simulink model "model_schuettgut"  (R2020a)
settings: Solver=VariableStepAuto  StartTime=0.0  StopTime=600  MaxStep=1e-2  MinStep=1e-5  RelTol=1e-2
libraries: simulink x8, library_schuettgut x5
settings Model: Creator=Jonathan  LastModifiedBy=Jonathan
settings DataIOCC: SaveState=on

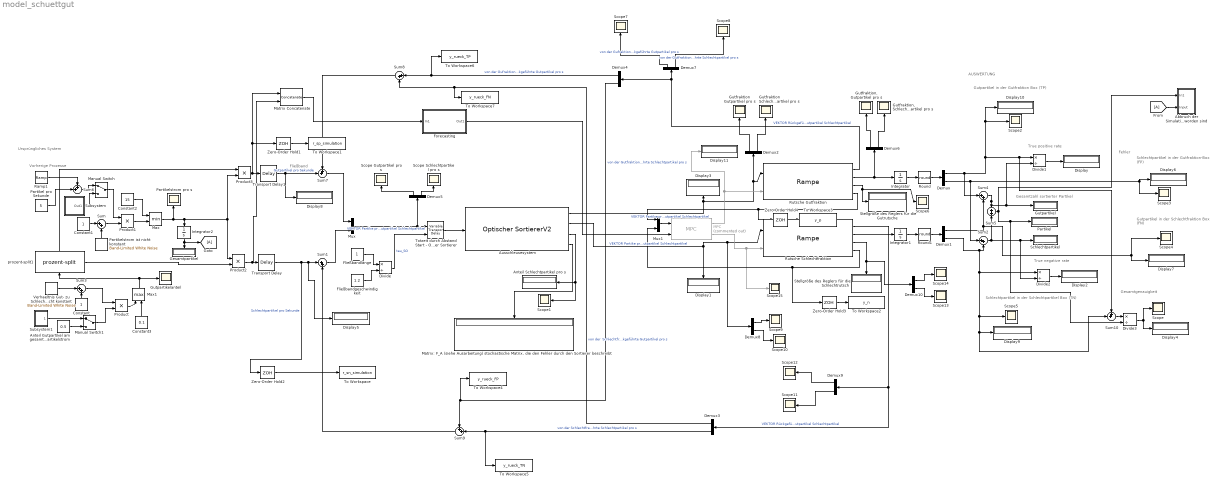
== system model_schuettgut ==
  note: Fließband
  note: Vorherige Prozesse
  note: Gesamtgenauigkeit
  note: True negative rate
  note: Gutpartikel in der
      | Schlechtfraktion Box (FN)
  note: Schlechtpartikel in der
      | Gutfraktion-Box (FP)
  note: Schlechtpartikel in der
      | Schlechtpartikel Box (TN)
  note: AUSWERTUNG
  note: True positive rate
  note: Gesamtzahl sortierter Partikel
  note: Gutpartikel in der
      | Gutfraktion Box (TP)
  note: Fehler
  note: Ursprüngliches System
  Abbruch der Simulation sobald alle Partikel sortiert worden sind : Subsystem
  Anteil Gutpartikel am gesamten Partikelstrom : Constant  Value=0.5
  Anteil Schlechtpartikel pro s : Display
  Ausschleusesystem : library_schuettgut/Optischer SortiererV2  alpha=0.04  beta=0.05
  Constant : Constant
  Constant1 : Constant
  Constant2 : Constant  Value=15
  Constant3 : Constant  Value=0.1
  Demux{,1..10} (11 alike) : Demux  Outputs=2
  Display{,1..11} (12 alike) : Display
  Divide{,1..3} (4 alike) : Product  Inputs=*/
  Fließbandgeschwindigkeit : Constant  Value=1.2
  Fließbandlänge : Constant
  Forecasting : Subsystem
  Gesamtpartikel : Display
  Gutfraktion Gutpartikel pro s : Scope
  Gutfraktion Schlechtpartikel pro s : Scope
  "Gutfraktion, Gutpartikel pro s" : Scope
  "Gutfraktion, Schlechtpartikel pro s" : Scope
  Gutpartikel : Display
  Gutpartikelanteil : Scope
  Integrator : Integrator
  Integrator1 : Integrator
  Integrator2 : Integrator
  MPC : library_schuettgut/MPC  Commented=on  SystemSampleTime=-1  Latency=0  AutoFrameSizeCalculation=off
      link override Constant: Value=12
      link override Constant2: Value=1
      link override Constant3: Value=4
      link override Constant4: Value=20
      link override Constant5: Value=8
      link override Constant6: Value=zeros(4,12)
  Manual Switch : ManualSwitch
  Manual Switch1 : ManualSwitch
  Matrix Concatenate : Concatenate  Mode=Multidimensional array  ConcatenateDimension=2
  "Matrix: F_A (siehe Ausarbeitung) stochastische Matrix, die den Fehler durch den Sortierer beschreibt" : Display
  Max : MinMax  Inputs=2
  Max1 : MinMax  Function=max  Inputs=2
  Mux : Mux  Inputs=2
  Mux1 : Mux  Inputs=2
  Partikel : Display
  Partikel pro Sekunde : Constant  Value=5
  Partikelstrom ist nicht konstant : simulink/Sources/Band-Limited White Noise  Cov=[0.00001]  Ts=0.1  seed=[23341]
  Partikelstrom pro s : Scope
  Product{,1..3} (4 alike) : Product
  Ramp1 : simulink/Sources/Ramp  slope=0.01  start=200  InitialOutput=0
  Round : Rounding  Operator=round
  Round1 : Rounding  Operator=round
  Rutsche Gutfraktion : library_schuettgut/Rampe  Tag=Rampe  OK=2  errorP=0  errorN=0  KV=0.2  V=1  TrueorFalse=0  delay=0.2  gain=8.6  KP=0  KN=0
  Rutsche Schlechtfraktion : library_schuettgut/Rampe  Tag=Rampe  OK=2  errorP=0  errorN=0  KV=0.2  V=1  TrueorFalse=1  delay=0.2  gain=0  KP=0  KN=0
  Schlechtpartikel : Display
  Scope{,1..15} (16 alike) : Scope
  Scope Gutpartikel pro s : Scope
  Scope Schlechtpartikel pro s : Scope
  Stellgröße des Reglers für die Gutrutsche : Display
  Stellgröße des Reglers für die Schlechtrutsch : Display
  Subsystem : Subsystem
  Subsystem1 : Subsystem
  Sum{,1..4,8} (6 alike) : Sum  Inputs=|++
  Sum{6..7,9..10} (4 alike) : Sum  Inputs=++|
  Sum5 : Sum  Inputs=+|+
  To Workspace : ToWorkspace  VariableName=r_sn_simulation  SaveFormat=Timeseries  SampleTime=-1
  To Workspace1 : ToWorkspace  VariableName=r_sp_simulation  SaveFormat=Timeseries  SampleTime=-1
  To Workspace2 : ToWorkspace  VariableName=y_n  SaveFormat=Timeseries  SampleTime=-1
  To Workspace3 : ToWorkspace  VariableName=y_p  SaveFormat=Timeseries  SampleTime=-1
  To Workspace4 : ToWorkspace  VariableName=y_rueck_FP  SaveFormat=Timeseries  SampleTime=0.1
  To Workspace5 : ToWorkspace  VariableName=y_rueck_TN  SaveFormat=Timeseries  SampleTime=0.1
  To Workspace6 : ToWorkspace  VariableName=y_rueck_TP  SaveFormat=Timeseries  SampleTime=0.1
  To Workspace7 : ToWorkspace  VariableName=y_rueck_FN  SaveFormat=Timeseries  SampleTime=0.1
  Totzeit durch Abstand Start - Optischer Sortierer : VariableTransportDelay  VariableDelayType=Variable transport delay  MaximumDelay=10  MaximumPoints=30000
  Transport Delay : TransportDelay  DelayTime=160  BufferSize=4096
  Transport Delay1 : TransportDelay  DelayTime=160  BufferSize=2048
  Verhaeltnis Gut- zu Schlechtpartikel ist nicht konstant : simulink/Sources/Band-Limited White Noise  Cov=[0.00001]  Ts=0.1  seed=[13341]
  Zero-Order Hold{1..4} (4 alike) : ZeroOrderHold  SampleTime=0.1
  prozent-split1 : library_schuettgut/prozent-split  SystemSampleTime=-1  Latency=0  AutoFrameSizeCalculation=off
      settings: PortSchema="{\"entries\":[{\"content\":{\"sides\":[{\"content\":{\"connectorIds\":[\"In1\"]},\"type\":\"ConnectorPlacement.EquallySpacedRectSide\",\"uuid\":\"ab8511c8-9f1d-48ad-bf24-85fd477f0bdd\"},{\"content\":{\"connectorIds\":[\"Out1\"],\"side\":\"RIGHT\"},\"type\":\"ConnectorPlacement.EquallySpacedRectSide\",\"uuid\":\"9ac1a19a-8176-444e-9f4d-7beffa0184e3\"},{\"content\":{\"connectorIds\":[\"Out2\"],\"side\":\"TOP\"},\"type\":\"ConnectorPlacement.EquallySpacedRectSide\",\"uuid\":\"376c2400-f821-4649-ab16-706a2da6117b\"}]},\"type\":\"ConnectorPlacement.EquallySpacedConnector\",\"uuid\":\"f6e72b2d-0467-4732-a018-d51f3a5db703\"}],\"packageUris\":[\"http://schema.mathworks.com/mf0/Connector/19700101\"],\"version\":\"1.0\"}"
  wires:
  Anteil Gutpartikel am gesamten Partikelstrom/1 -> Manual Switch1/2
  Max/1 -> Partikelstrom pro s/1, Integrator2/1, Product2/1, Product3/2
  Transport Delay1/1 -> Display8/1, Sum7/2  "Gutpartikel pro Sekunde"
  Totzeit durch Abstand Start - Optischer Sortierer/1 -> Ausschleusesystem/1
  Rutsche Gutfraktion/1 -> Demux4/1, Demux7/1  "VEKTOR Rückgeführte Partikel Gutfraktion pro s Gutpartikel Schlechtpartikel"
  Mux/1 -> Totzeit durch Abstand Start - Optischer Sortierer/1, Demux5/1  "VEKTOR Partike pro s: Gutpartikel Schlechtpartikel"
  Demux4/1 -> To Workspace6/1, Sum8/1  "von der Gufraktion zurückgeführte Gutpartikel pro s"
  Sum8/1 -> Sum7/1
  Sum9/1 -> Sum1/2
  Rutsche Gutfraktion/2 -> Demux6/1, Integrator/1
  Ausschleusesystem/1 -> Demux2/1, Rutsche Gutfraktion/1, Display3/1  "VEKTOR Partike pro s in der Gutfraktion: Gutpartikel Schlechtpartikel"
  Ausschleusesystem/2 -> Display1/1, Demux8/1, Rutsche Schlechtfraktion/1  "VEKTOR Partike pro s in der Schlechtfraktion: Gutpartikel Schlechtpartikel"
  Max1/1 -> prozent-split1/1, Gutpartikelanteil/1
  prozent-split1/1 -> Product3/1
  prozent-split1/2 -> Product2/2
  Product2/1 -> Matrix Concatenate/2, Transport Delay/1
  Sum1/1 -> Mux/2
  Sum7/1 -> Mux/1
  Demux3/2 -> To Workspace5/1, Sum9/2  "von der Schlechtfraktion zurückgeführte Schlechtpartikel pro s"
  Demux4/2 -> To Workspace4/1, Sum9/1  "von der Gutfraktion zurückgeführte Schlechtpartikel pro s"
  Demux3/1 -> To Workspace7/1, Sum8/2  "von der  Schlechtfraktion zurückgeführte Gutpartikel pro s"
  Demux/1 -> Sum4/1, Display10/1, Scope2/1, Sum10/1, Divide1/1
  Demux/2 -> Display6/1, Scope3/1, Sum2/1
  Demux1/1 -> Sum4/2, Scope4/1, Display7/1
  Demux1/2 -> Divide2/1, Sum10/2, Display9/1, Scope5/1, Sum2/2
  Rutsche Schlechtfraktion/2 -> Integrator1/1
  Integrator/1 -> Round/1
  Integrator1/1 -> Round1/1
  Demux2/2 -> Gutfraktion Schlechtpartikel pro s/1
  Demux2/1 -> Gutfraktion Gutpartikel pro s/1
  Rutsche Schlechtfraktion/1 -> Demux9/1, Demux3/1  "VEKTOR Rückgeführte Partikel Schlechtfraktion pro s Gutpartikel Schlechtpartikel"
  Ausschleusesystem/3 -> Scope1/1, Anteil Schlechtpartikel pro s/1
  Demux5/1 -> Scope Gutpartikel pro s/1
  Demux5/2 -> Scope Schlechtpartikel pro s/1
  Divide/1 -> Totzeit durch Abstand Start - Optischer Sortierer/2  "tau_SO"
  Fließbandgeschwindigkeit/1 -> Divide/2
  Fließbandlänge/1 -> Divide/1
  Round/1 -> Demux/1
  Round1/1 -> Demux1/1
  Sum3/1 -> Product/1
  Constant/1 -> Sum3/2
  Demux6/1 -> "Gutfraktion, Gutpartikel pro s"/1
  Demux6/2 -> "Gutfraktion, Schlechtpartikel pro s"/1
  Constant1/1 -> Sum/1
  Sum/1 -> Product1/2
  Ausschleusesystem/4 -> "Matrix: F_A (siehe Ausarbeitung) stochastische Matrix, die den Fehler durch den Sortierer beschreibt"/1
  Rutsche Gutfraktion/3 -> Stellgröße des Reglers für die Gutrutsche/1, Scope6/1
  Rutsche Schlechtfraktion/3 -> Demux10/1, Stellgröße des Reglers für die Schlechtrutsch/1
  Verhaeltnis Gut- zu Schlechtpartikel ist nicht konstant/1 -> Sum3/1
  Constant2/1 -> Max/1
  Manual Switch/1 -> Product1/1
  Partikelstrom ist nicht konstant/1 -> Sum/2
  Integrator2/1 -> [A], Gesamtpartikel/1
  Sum2/1 -> Divide2/2, Schlechtpartikel/1, Sum5/2
  Sum4/1 -> Divide1/2, Gutpartikel/1, Sum5/1
  Sum5/1 -> Partikel/1, Divide3/2, Abbruch der Simulation sobald alle Partikel sortiert worden sind/1(In1)
  Subsystem/1(Out1) -> Manual Switch/2
  Partikel pro Sekunde/1 -> Sum6/2
  Subsystem1/1(Out1) -> Manual Switch1/1
  Manual Switch1/1 -> Product/2
  Divide1/1 -> Display/1
  [A] -> Abbruch der Simulation sobald alle Partikel sortiert worden sind/2(Input)
  Divide2/1 -> Display2/1
  Product1/1 -> Max/2
  Product/1 -> Max1/1
  Constant3/1 -> Max1/2
  Ramp1/1 -> Sum6/1
  Sum6/1 -> Manual Switch/1
  Demux7/1 -> Scope7/1  "von der Gufraktion zurückgeführte Gutpartikel pro s"
  Demux7/2 -> Scope8/1  "von der Gutfraktion zurückgeführte Schlechtpartikel pro s"
  Sum10/1 -> Divide3/1
  Divide3/1 -> Display4/1, Scope/1
  MPC/1 -> Rutsche Gutfraktion/2, Display11/1
  MPC/2 -> Scope15/1, Rutsche Schlechtfraktion/2
  Mux1/1 -> MPC/1
  Rutsche Schlechtfraktion/4 -> Zero-Order Hold3/1, Mux1/2
  Rutsche Gutfraktion/4 -> Zero-Order Hold4/1, Mux1/1
  Product3/1 -> Matrix Concatenate/1, Zero-Order Hold1/1, Transport Delay1/1
  Zero-Order Hold1/1 -> To Workspace1/1
  Zero-Order Hold2/1 -> To Workspace/1
  Transport Delay/1 -> Zero-Order Hold2/1, Display5/1, Sum1/1  "Schlechtpartikel pro Sekunde"
  Matrix Concatenate/1 -> Forecasting/1(In1)
  Forecasting/1(Out1) -> MPC/2
  Demux8/2 -> Scope10/1
  Demux8/1 -> Scope9/1
  Demux9/1 -> Scope12/1
  Demux9/2 -> Scope11/1
  Demux10/1 -> Scope14/1
  Demux10/2 -> Scope13/1
  Zero-Order Hold3/1 -> To Workspace2/1
  Zero-Order Hold4/1 -> To Workspace3/1

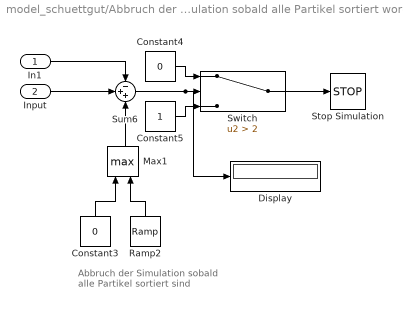
== system model_schuettgut/Abbruch der Simulation sobald alle Partikel sortiert worden sind ==
  note: Abbruch der Simulation sobald
      | alle Partikel sortiert sind
  In1 : Inport
  Input : Inport  Port=2
  Constant3 : Constant  Value=0
  Constant4 : Constant  Value=0
  Constant5 : Constant
  Display : Display
  Max1 : MinMax  Function=max  Inputs=2
  Ramp2 : simulink/Sources/Ramp  slope=-1  start=50  InitialOutput=10
  Stop Simulation : Stop
  Sum6 : Sum  Inputs=-++
  Switch : Switch  Criteria=u2 > Threshold  Threshold=2
  wires:
  Input/1 -> Sum6/2
  Constant4/1 -> Switch/1
  Switch/1 -> Stop Simulation/1
  Constant5/1 -> Switch/3
  Ramp2/1 -> Max1/2
  Sum6/1 -> Display/1, Switch/2
  Constant3/1 -> Max1/1
  Max1/1 -> Sum6/3
  In1/1 -> Sum6/1

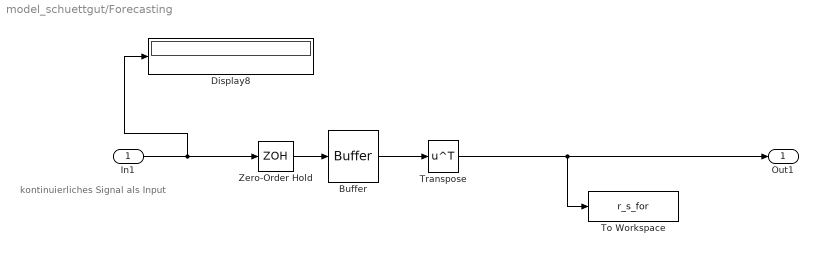
== system model_schuettgut/Forecasting ==
  note: kontinuierliches Signal als Input
  In1 : Inport
  Buffer : Buffer  N=400  V=399  OutputFrames=off
  Display8 : Display
  To Workspace : ToWorkspace  VariableName=r_s_for  SaveFormat=Timeseries  SampleTime=0.4
  Transpose : Math  Operator=transpose  SaturateOnIntegerOverflow=on
  Zero-Order Hold : ZeroOrderHold  SampleTime=0.4
  Out1 : Outport
  wires:
  Buffer/1 -> Transpose/1
  In1/1 -> Display8/1, Zero-Order Hold/1
  Zero-Order Hold/1 -> Buffer/1
  Transpose/1 -> To Workspace/1, Out1/1

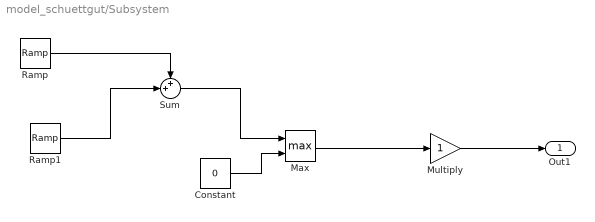
== system model_schuettgut/Subsystem ==
  Constant : Constant  Value=0
  Max : MinMax  Function=max  Inputs=2
  Multiply : Gain
  Ramp : simulink/Sources/Ramp  slope=10  start=0  InitialOutput=0
  Ramp1 : simulink/Sources/Ramp  slope=-20  start=100  InitialOutput=0
  Sum : Sum  Inputs=++|
  Out1 : Outport
  wires:
  Max/1 -> Multiply/1
  Constant/1 -> Max/2
  Sum/1 -> Max/1
  Ramp1/1 -> Sum/2
  Ramp/1 -> Sum/1
  Multiply/1 -> Out1/1

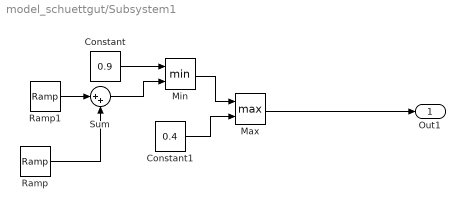
== system model_schuettgut/Subsystem1 ==
  Constant : Constant  Value=0.9
  Constant1 : Constant  Value=0.4
  Max : MinMax  Function=max  Inputs=2
  Min : MinMax  Inputs=2
  Ramp : simulink/Sources/Ramp  slope=0.01  start=20  InitialOutput=0.7
  Ramp1 : simulink/Sources/Ramp  slope=-0.03  start=150  InitialOutput=0
  Sum : Sum  Inputs=|++
  Out1 : Outport
  wires:
  Max/1 -> Out1/1
  Constant/1 -> Min/1
  Constant1/1 -> Max/2
  Min/1 -> Max/1
  Sum/1 -> Min/2
  Ramp1/1 -> Sum/1
  Ramp/1 -> Sum/2
